simulink model "deedemo2"  (Simulink 3.00)
settings: Solver=ode45  SolverMode=SingleTasking  StartTime=0.0  StopTime=999999  RelTol=1e-3  AbsTol=1e-6
PreLoadFcn:
  | lorenzi
undefined symbols (not defined in the file or in its folder): beta, rho, sigma
libraries: simulink3 x1
settings Model: SaveTime=off  SaveOutput=off  Creator=sanjai  LastModifiedBy=sanjai

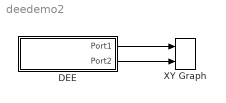
== system deedemo2 ==
  DEE : Subsystem
      settings: OpenFcn=diffeqed
      mask Type: Differential Equation Editor (DEE)
      mask Display: disp('Lorenz Attractor')
  XY Graph : simulink3/Sinks/XY Graph  xmin=-30  xmax=30  ymin=0  ymax=50  st=0.025
  wires:
  DEE/2(Port2) -> XY Graph/2
  DEE/1(Port1) -> XY Graph/1

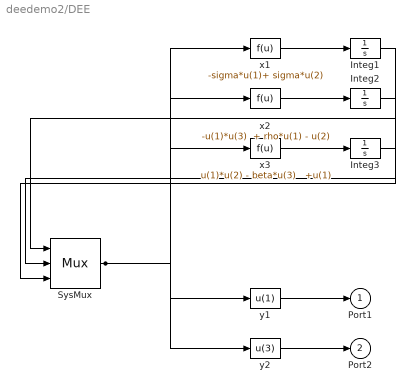
== system deedemo2/DEE ==
  Integ1 : Integrator  ExternalReset=none  InitialConditionSource=internal  InitialCondition=1  LimitOutput=off  UpperSaturationLimit=inf  LowerSaturationLimit=-inf  ShowSaturationPort=off  ShowStatePort=off  AbsoluteTolerance=auto
  Integ2 : Integrator  ExternalReset=none  InitialConditionSource=internal  InitialCondition=1  LimitOutput=off  UpperSaturationLimit=inf  LowerSaturationLimit=-inf  ShowSaturationPort=off  ShowStatePort=off  AbsoluteTolerance=auto
  Integ3 : Integrator  ExternalReset=none  InitialConditionSource=internal  InitialCondition=1  LimitOutput=off  UpperSaturationLimit=inf  LowerSaturationLimit=-inf  ShowSaturationPort=off  ShowStatePort=off  AbsoluteTolerance=auto
  SysMux : Mux  Inputs=3
      settings: DisplayOption=none
  x1 : Fcn  Expr=-sigma*u(1)+ sigma*u(2)
  x2 : Fcn  Expr="-u(1)*u(3)  + rho*u(1) - u(2)"
  x3 : Fcn  Expr="u(1)*u(2) - beta*u(3)   +u(1)"
  y1 : Fcn  Expr=u(1)
  y2 : Fcn  Expr=u(3)
  Port1 : Outport  Port=1  InitialOutput=0
  Port2 : Outport  Port=2  InitialOutput=0
  wires:
  y2/1 -> Port2/1
  SysMux/1 -> y2/1, y1/1, x3/1, x2/1, x1/1
  y1/1 -> Port1/1
  Integ3/1 -> SysMux/3
  x3/1 -> Integ3/1
  Integ2/1 -> SysMux/2
  x2/1 -> Integ2/1
  Integ1/1 -> SysMux/1
  x1/1 -> Integ1/1
